simulink model "Jumping_Spherical_System"  (R2023a)
settings: Solver=VariableStepAuto  StartTime=0.0  StopTime=simtime  MaxStep=0.01  RelTol=1e-3
undefined symbols (not defined in the file): c, g, h_0, k_AR, m
settings Model: Creator=fycce  LastModifiedBy=fycce
settings DataIOCC: SaveOutput=off  SaveTime=off  ReturnWorkspaceOutputs=off

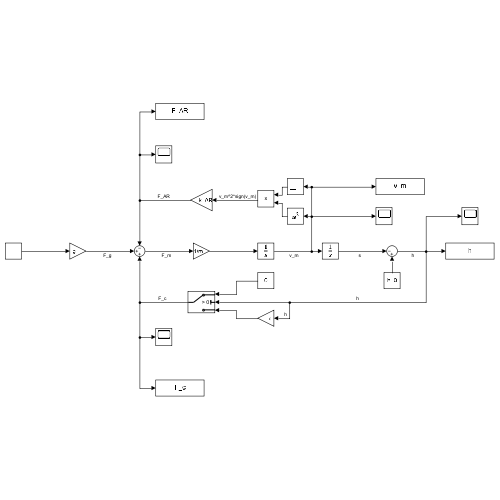
[thumbnail: Simulink's stored preview of the top-level diagram]
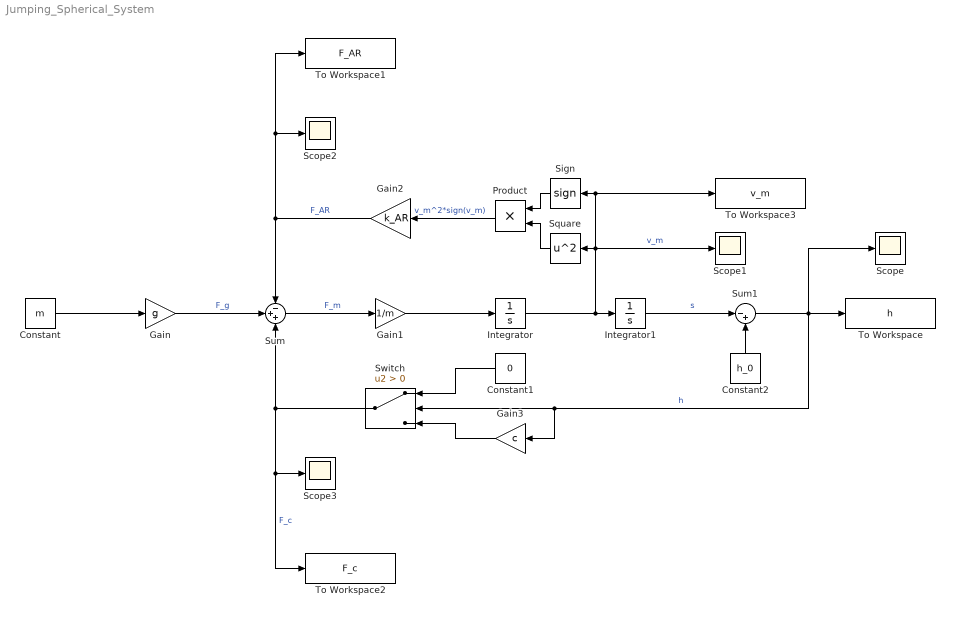
== system Jumping_Spherical_System ==
  Constant : Constant  Value=m
  Constant1 : Constant  Value=0
  Constant2 : Constant  Value=h_0
  Gain : Gain  Gain=g
  Gain1 : Gain  Gain=1/m
  Gain2 : Gain  Gain=k_AR
  Gain3 : Gain  Gain=c
  Integrator : Integrator
  Integrator1 : Integrator
  Product : Product
  Scope{,1..3} (4 alike) : Scope
  Sign : Signum
  Square : Math  Operator=square
  Sum : Sum  Inputs=-++
  Sum1 : Sum  Inputs=|-+
  Switch : Switch  Criteria=u2 > Threshold  SaturateOnIntegerOverflow=off  InputSameDT=off
  To Workspace : ToWorkspace  VariableName=h  SaveFormat=Timeseries  SampleTime=-1
  To Workspace1 : ToWorkspace  VariableName=F_AR  SaveFormat=Timeseries  SampleTime=-1
  To Workspace2 : ToWorkspace  VariableName=F_c  SaveFormat=Timeseries  SampleTime=-1
  To Workspace3 : ToWorkspace  VariableName=v_m  SaveFormat=Timeseries  SampleTime=-1
  wires:
  Constant/1 -> Gain/1
  Gain/1 -> Sum/2  "F_g"
  Sum/1 -> Gain1/1  "F_m"
  Gain2/1 -> To Workspace1/1, Scope2/1, Sum/1  "F_AR"
  Product/1 -> Gain2/1  "v_m^2*sign(v_m)"
  Gain1/1 -> Integrator/1
  Integrator/1 -> Scope1/1, To Workspace3/1, Sign/1, Square/1, Integrator1/1  "v_m"
  Sign/1 -> Product/1
  Integrator1/1 -> Sum1/1  "s"
  Constant2/1 -> Sum1/2
  Sum1/1 -> Switch/2, Gain3/1, To Workspace/1, Scope/1  "h"
  Square/1 -> Product/2
  Switch/1 -> To Workspace2/1, Scope3/1, Sum/3  "F_c"
  Gain3/1 -> Switch/3
  Constant1/1 -> Switch/1
